simulink model "Project_1_8"  (R2016b)
settings: Solver=ode45  StartTime=0.0  StopTime=1  RelTol=1e-3  EnableMultiTasking=on
values from neighbouring files (symbols this model uses):
  A = [A_zero I; -inv(M)*K -inv(M)*D]    [Final_Project_JustinGarcia.m]    (also in Final_Project_Justin_Garcia_190.m = [A_zero initial; -inv(M)*K_equation -inv(M)*D]; projectpart1.m = [zeros(2,2) [1 0;0 1] ; -inv(M)*K -inv(M)*D])
  B = [B_zero;inv(M)*F]    [Final_Project_JustinGarcia.m]    (also in Final_Project_Justin_Garcia_190.m; projectpart1.m = [zeros(2,1); inv(M)*F])
settings Model: Creator=009759399  LastModifiedBy=Mac
settings DataIOCC: LimitDataPoints=on  SaveFormat=Array
settings OptimizationCC: LifeSpan=inf
settings DebuggingCC: SFUnexpectedBacktrackingDiag=warning  SFNoUnconditionalDefaultTransitionDiag=warning  SFExecutionAtInitializationDiag=none
settings HardwareCC: ProdBitPerPointer=32  ProdBitPerSizeT=32  ProdBitPerPtrDiffT=32  ProdLargestAtomicFloat=None  ProdIntDivRoundTo=Undefined  ProdEndianess=Unspecified  ProdWordSize=32  ProdHWDeviceType=32-bit Generic
settings ModelReferenceCC: PropagateSignalLabelsOutOfModel=off
settings GRTTargetCC: TargetLangStandard=C89/C90 (ANSI)  GeneratePreprocessorConditionals=Disable all
settings ConfigComp: CovMetricSettings=dw  CovHtmlReporting=on  CovSaveCumulativeToWorkspaceVar=on  CovSaveSingleToWorkspaceVar=on  CovExternalEMLEnable=off

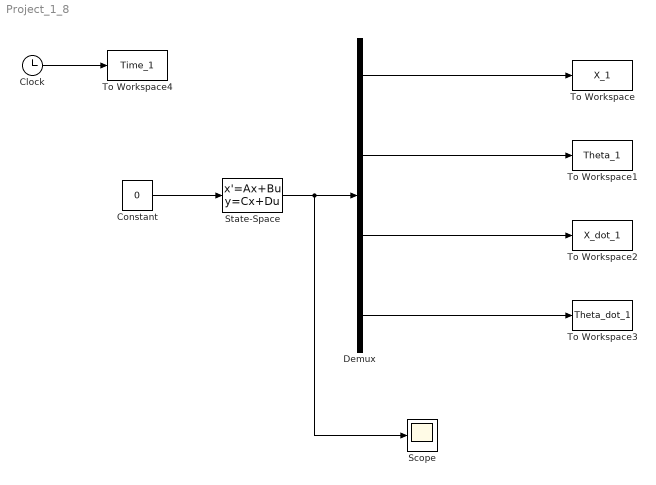
== system Project_1_8 ==
  Clock : Clock
  Constant : Constant  Value=0
  Demux : Demux
  Scope : Scope
  State-Space : StateSpace  A=A  B=B  C=[1 0 0 0;0 1 0 0; 0 0 1 0; 0 0 0 1]  D=[0;0;0;0]  X0=[0;pi/60;0;0]
  To Workspace : ToWorkspace  VariableName=X_1  SampleTime=-1
  To Workspace1 : ToWorkspace  VariableName=Theta_1  SampleTime=-1
  To Workspace2 : ToWorkspace  VariableName=X_dot_1  SampleTime=-1
  To Workspace3 : ToWorkspace  VariableName=Theta_dot_1  SampleTime=-1
  To Workspace4 : ToWorkspace  VariableName=Time_1  SampleTime=-1
  wires:
  Constant/1 -> State-Space/1
  State-Space/1 -> Scope/1, Demux/1
  Demux/1 -> To Workspace/1
  Demux/2 -> To Workspace1/1
  Demux/3 -> To Workspace2/1
  Demux/4 -> To Workspace3/1
  Clock/1 -> To Workspace4/1
